simulink model "FullAdder"  (R2023a)
settings: Solver=VariableStepAuto  StartTime=0.0  StopTime=1  RelTol=1e-3
settings Model: Creator=Admin  LastModifiedBy=Admin

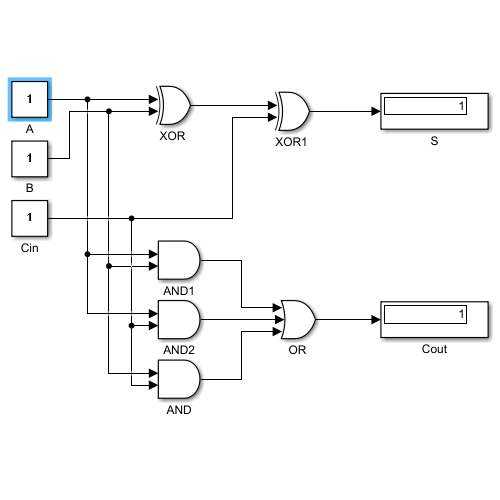
[thumbnail: Simulink's stored preview of the top-level diagram]
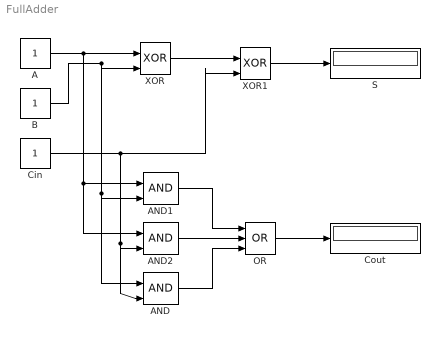
== system FullAdder ==
  A : Constant  SampleTime=-1
  AND : Logic  IconShape=distinctive  AllPortsSameDT=off  OutDataTypeStr=boolean
  AND1 : Logic  IconShape=distinctive  AllPortsSameDT=off  OutDataTypeStr=boolean
  AND2 : Logic  IconShape=distinctive  AllPortsSameDT=off  OutDataTypeStr=boolean
  B : Constant  SampleTime=-1
  Cin : Constant  SampleTime=-1
  Cout : Display
  OR : Logic  Operator=OR  Inputs=3  IconShape=distinctive  AllPortsSameDT=off  OutDataTypeStr=boolean
  S : Display
  XOR : Logic  Operator=XOR  IconShape=distinctive  AllPortsSameDT=off  OutDataTypeStr=boolean
  XOR1 : Logic  Operator=XOR  IconShape=distinctive  AllPortsSameDT=off  OutDataTypeStr=boolean
  wires:
  A/1 -> AND2/1, AND1/1, XOR/1
  B/1 -> AND/1, AND1/2, XOR/2
  XOR/1 -> XOR1/1
  Cin/1 -> AND2/2, AND/2, XOR1/2
  AND2/1 -> OR/2
  AND1/1 -> OR/1
  AND/1 -> OR/3
  XOR1/1 -> S/1
  OR/1 -> Cout/1
